simulink model "nav_flocking33"  (R2022b)
settings: Solver=FixedStepAuto  StartTime=0.0  StopTime=10.0  FixedStep=0.01  RelTol=1e-3
values from neighbouring files (symbols this model uses):
  a = 1    [main_flock3.m]    (also in main_flock4.m; params_flocking_ros.m)
  aR = diag([ar; ap; ay])    [main_flock3.m]    (also in main_flock4.m; main_sliding.m)
  Att1 = [2 -2 -15]    [main_flock3.m]    (also in main_flock4.m)
  Att2 = [2 -2 -15]    [main_flock3.m]    (also in main_flock4.m)
  Att3 = [2 -2 -15]    [main_flock3.m]    (also in main_flock4.m)
  b = 1    [main_flock3.m]    (also in main_flock4.m; params_flocking_ros.m)
  c = 1    [main_flock3.m]    (also in main_flock4.m; params_flocking_ros.m)
  c_gammap = 1.2    [main_flock3.m]    (also in main_flock4.m)
  c_gammav = 3.5    [main_flock3.m]    (also in main_flock4.m)
  d = 0.6    [main_flock3.m]    (also in main_flock4.m; params_flocking_ros.m)
  d_prime = 1    [main_flock3.m]    (also in main_flock4.m; params_flocking_ros.m)
  epsilon = 0.1    [main_flock3.m]    (also in main_flock4.m; params_flocking_ros.m)
  h = 0.2    [main_flock3.m]    (also in main_flock4.m; params_flocking_ros.m)
  K1 = diag([k111; k122; k133])    [main_flock3.m]    (also in main_flock4.m; main_sliding.m)
  K2 = diag([k211; k222; k233])    [main_flock3.m]    (also in main_flock4.m; main_sliding.m)
  Ki = diag([Ki1; Ki2; Ki3])    [main_flock3.m]    (also in main_flock4.m; main_sliding.m)
  lam = diag([lam1; lam2; lam3])    [main_flock3.m]    (also in main_flock4.m; main_sliding.m)
  R = 0.15    [main_flock3.m]    (also in main_flock4.m; params_flocking_ros.m)
  vxobs = 0    [main_flock3.m]    (also in main_flock4.m)
  vyobs = 0    [main_flock3.m]    (also in main_flock4.m)
  vzobs = 0    [main_flock3.m]    (also in main_flock4.m)
  X0_1 = [P01 dP01 om01]    [main_flock3.m]    (also in main_flock4.m; main_sliding.m = [P0 dP0 om0])
  X0_2 = [P02 dP02 om02]    [main_flock3.m]    (also in main_flock4.m)
  X0_3 = [P03 dP03 om03]    [main_flock3.m]    (also in main_flock4.m)
  xmax = 2    [main_flock3.m]    (also in main_flock4.m)
  xmin = -2    [main_flock3.m]    (also in main_flock4.m)
  xobs = 0.75    [main_flock3.m]    (also in main_flock4.m)
  yobs = -0.25    [main_flock3.m]    (also in main_flock4.m)
  zobs = 1.7    [main_flock3.m]    (also in main_flock4.m)
undefined symbols (not defined in the file or in its folder): A_Euler
libraries: aerosimlib x3
(part 1 of 2)
settings Model: Creator=root  LastModifiedBy=jonatan_alvarez
settings SolverCC: AlgebraicLoopSolver=TrustRegion
settings DataIOCC: ReturnWorkspaceOutputs=off
settings DebuggingCC: UnconnectedInputMsg=warning  UnconnectedOutputMsg=warning  UnconnectedLineMsg=warning  SFMachineParentedDataDiag=warning  UnderSpecifiedDimensionMsg=warning  ArithmeticOperatorsInVariantConditions=warning
settings ModelReferenceCC: EnableRefExpFcnMdlSchedulingChecks=on
settings SFSimCC: CustomCodeUndefinedFunction=UseInterfaceOnly

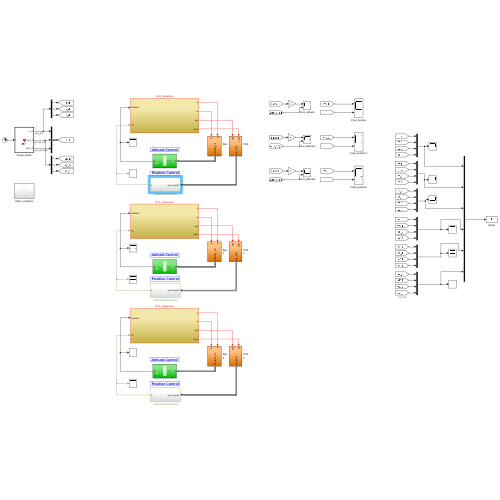
[thumbnail: Simulink's stored preview of the top-level diagram]
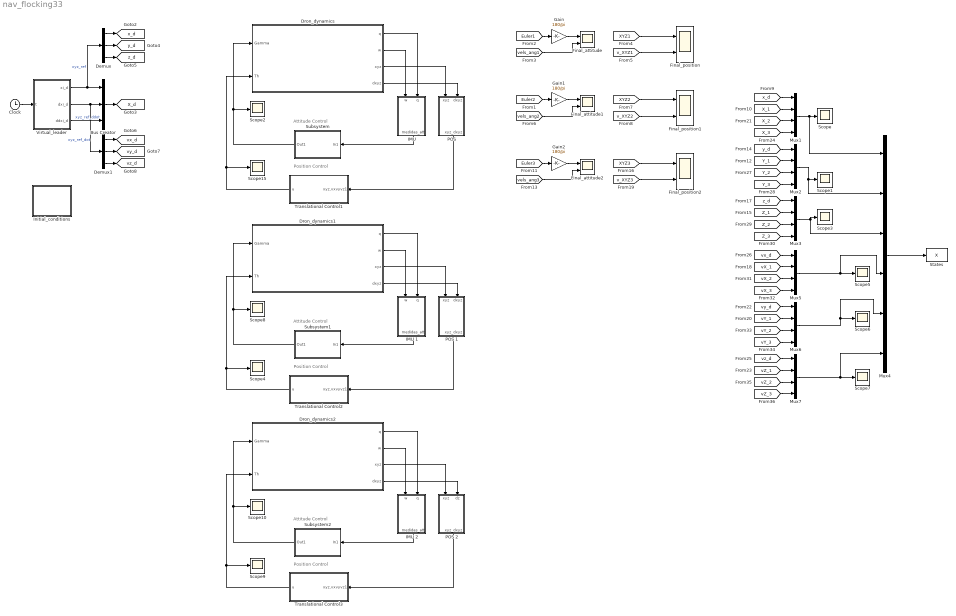
== system nav_flocking33 ==
  note: Position Control
  note: Attitude Control
  note: Position Control
  note: Attitude Control
  note: Position Control
  note: Attitude Control
  Bus Creator : BusCreator  Inputs=3
  Clock : Clock
  Demux : Demux  Outputs=3
  Demux1 : Demux  Outputs=3
  Dron_dynamics : Subsystem
  Dron_dynamics1 : Subsystem
  Dron_dynamics2 : Subsystem
  Final_attitude : Scope  NumInputPorts=2
  Final_attitude1 : Scope  NumInputPorts=2
  Final_attitude2 : Scope  NumInputPorts=2
  Final_position : Scope  NumInputPorts=2
  Final_position1 : Scope  NumInputPorts=2
  Final_position2 : Scope  NumInputPorts=2
  Gain : Gain  Gain=180/pi
  Gain1 : Gain  Gain=180/pi
  Gain2 : Gain  Gain=180/pi
  "IMU " : Subsystem
  IMU 1 : Subsystem
  IMU 2 : Subsystem
  Initial_conditions : Subsystem
  Mux{1..3,5..7} (6 alike) : Mux
  Mux4 : Mux  Inputs=6
  "POS " : Subsystem
  POS 1 : Subsystem
  POS 2 : Subsystem
  Scope{,1..10,15} (12 alike) : Scope
  States : ToWorkspace  VariableName=X  SampleTime=-1
  Subsystem : Subsystem
  Subsystem1 : Subsystem
  Subsystem2 : Subsystem
  Translational Control1 : Subsystem
  Translational Control2 : Subsystem
  Translational Control3 : Subsystem
  Virtual_leader : MATLAB Function  TreatAsAtomicUnit=on
  tag scope: X_d=global, vx_d=global, vy_d=global, vz_d=global, x_d=global, y_d=global, z_d=global
  wires:
  [vels_ang1] -> Final_attitude/2
  [v_XYZ1] -> Final_position/2
  Gain/1 -> Final_attitude/1
  [XYZ1] -> Final_position/1
  [Euler1] -> Gain/1
  Dron_dynamics/2(w) -> "IMU "/1(w)
  Dron_dynamics/4(dxyz) -> "POS "/2(dxyz)
  Bus Creator/1 -> [X_d]
  Virtual_leader/3(ddxi_d) -> Bus Creator/3  "xyz_ref_ddot"
  Dron_dynamics/1(q) -> "IMU "/2(q)
  Subsystem/1(Out1) -> Scope2/1, Dron_dynamics/1(Gamma)
  Dron_dynamics/3(xyz) -> "POS "/1(xyz)
  "POS "/1(xyz_dxyz) -> Translational Control1/1(xyz,vxvyvz1)
  Translational Control1/1(u) -> Scope15/1, Dron_dynamics/2(Th)
  "IMU "/1(medidas_att) -> Subsystem/1(In1)
  Virtual_leader/1(xi_d) -> Demux/1, Bus Creator/1  "xyz_ref"
  Demux/1 -> [x_d]
  Demux/2 -> [y_d]
  Demux/3 -> [z_d]
  [x_d] -> Mux1/1
  [X_1] -> Mux1/2
  Mux2/1 -> Mux4/2, Scope1/1
  [Y_1] -> Mux2/2
  [y_d] -> Mux2/1
  [z_d] -> Mux3/1
  [Z_1] -> Mux3/2
  Mux3/1 -> Scope3/1, Mux4/3
  Mux4/1 -> States/1
  Mux1/1 -> Mux4/1, Scope/1
  Demux1/3 -> [vz_d]
  Demux1/2 -> [vy_d]
  Demux1/1 -> [vx_d]
  Virtual_leader/2(dxi_d) -> Demux1/1, Bus Creator/2  "xyz_ref_dot"
  [vZ_1] -> Mux7/2
  [vz_d] -> Mux7/1
  [vy_d] -> Mux6/1
  [vY_1] -> Mux6/2
  [vX_1] -> Mux5/2
  [vx_d] -> Mux5/1
  Mux5/1 -> Scope5/1, Mux4/4
  Mux6/1 -> Scope6/1, Mux4/5
  Mux7/1 -> Mux4/6, Scope7/1
  Clock/1 -> Virtual_leader/1(t)
  Dron_dynamics1/2(w) -> IMU 1/1(w)
  Dron_dynamics1/4(dxyz) -> POS 1/2(dxyz)
  Dron_dynamics1/3(xyz) -> POS 1/1(xyz)
  POS 1/1(xyz_dxyz) -> Translational Control2/1(xyz,vxvyvz1)
  Dron_dynamics1/1(q) -> IMU 1/2(q)
  Translational Control2/1(u) -> Scope4/1, Dron_dynamics1/2(Th)
  IMU 1/1(medidas_att) -> Subsystem1/1(In1)
  Subsystem1/1(Out1) -> Scope8/1, Dron_dynamics1/1(Gamma)
  Dron_dynamics2/2(w) -> IMU 2/1(w)
  Dron_dynamics2/4(dxyz) -> POS 2/2(dz)
  Dron_dynamics2/3(xyz) -> POS 2/1(xyz)
  POS 2/1(xyz_dxyz) -> Translational Control3/1(xyz,vxvyvz1)
  Dron_dynamics2/1(q) -> IMU 2/2(q)
  Translational Control3/1(u) -> Scope9/1, Dron_dynamics2/2(Th)
  IMU 2/1(medidas_att) -> Subsystem2/1(In1)
  Subsystem2/1(Out1) -> Scope10/1, Dron_dynamics2/1(Gamma)
  [v_XYZ2] -> Final_position1/2
  [Euler2] -> Gain1/1
  Gain1/1 -> Final_attitude1/1
  [XYZ2] -> Final_position1/1
  [vels_ang2] -> Final_attitude1/2
  [v_XYZ3] -> Final_position2/2
  [Euler3] -> Gain2/1
  Gain2/1 -> Final_attitude2/1
  [XYZ3] -> Final_position2/1
  [vels_ang3] -> Final_attitude2/2
  [X_2] -> Mux1/3
  [X_3] -> Mux1/4
  [Y_2] -> Mux2/3
  [Y_3] -> Mux2/4
  [Z_2] -> Mux3/3
  [Z_3] -> Mux3/4
  [vX_2] -> Mux5/3
  [vX_3] -> Mux5/4
  [vY_2] -> Mux6/3
  [vY_3] -> Mux6/4
  [vZ_2] -> Mux7/3
  [vZ_3] -> Mux7/4

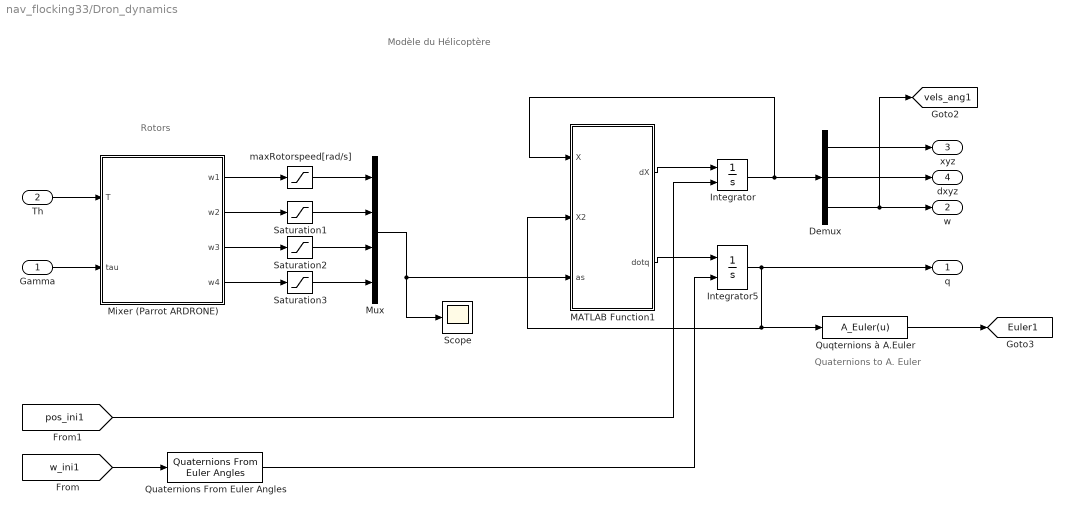
== system nav_flocking33/Dron_dynamics ==
  note: Modèle du Hélicoptère
  note: Rotors
  note: Quaternions to A. Euler
  Gamma : Inport
  Th : Inport  Port=2
  Demux : Demux  Outputs=3
  Integrator : Integrator  InitialConditionSource=external
  Integrator5 : Integrator  InitialConditionSource=external  InitialCondition=[1 0 0 0]
  MATLAB Function1 : MATLAB Function  TreatAsAtomicUnit=on
  Mixer (Parrot ARDRONE) : MATLAB Function  TreatAsAtomicUnit=on
  Mux : Mux
  Quaternions From Euler Angles : aerosimlib/Transformations/Quaternions From Euler Angles
  Quqternions à A.Euler : MATLABFcn  MATLABFcn=A_Euler(u)  OutputDimensions=3
  Saturation1 : Saturate  UpperLimit=1100  LowerLimit=5
  Saturation2 : Saturate  UpperLimit=1100  LowerLimit=5
  Saturation3 : Saturate  UpperLimit=1100  LowerLimit=5
  Scope : Scope
  maxRotorspeed[rad/s] : Saturate  UpperLimit=1100  LowerLimit=5
  q : Outport  VectorParamsAs1DForOutWhenUnconnected=off
  w : Outport  Port=2  VectorParamsAs1DForOutWhenUnconnected=off
  xyz : Outport  Port=3  VectorParamsAs1DForOutWhenUnconnected=off
  dxyz : Outport  Port=4  VectorParamsAs1DForOutWhenUnconnected=off
  tag scope: Euler1=global, vels_ang1=global
  wires:
  [w_ini1] -> Quaternions From Euler Angles/1
  Quqternions à A.Euler/1 -> [Euler1]
  Mixer (Parrot ARDRONE)/4(w4) -> Saturation3/1
  Saturation1/1 -> Mux/2
  Mixer (Parrot ARDRONE)/2(w2) -> Saturation1/1
  Mixer (Parrot ARDRONE)/1(w1) -> maxRotorspeed[rad/s]/1
  maxRotorspeed[rad/s]/1 -> Mux/1
  Saturation3/1 -> Mux/4
  Saturation2/1 -> Mux/3
  Mixer (Parrot ARDRONE)/3(w3) -> Saturation2/1
  Mux/1 -> Scope/1, MATLAB Function1/3(as)
  Integrator5/1 -> MATLAB Function1/2(X2), Quqternions à A.Euler/1, q/1
  MATLAB Function1/1(dX) -> Integrator/1
  MATLAB Function1/2(dotq) -> Integrator5/1
  Quaternions From Euler Angles/1 -> Integrator5/2
  Integrator/1 -> Demux/1, MATLAB Function1/1(X)
  Gamma/1 -> Mixer (Parrot ARDRONE)/2(tau)
  [pos_ini1] -> Integrator/2
  Demux/3 -> [vels_ang1], w/1
  Demux/1 -> xyz/1
  Demux/2 -> dxyz/1
  Th/1 -> Mixer (Parrot ARDRONE)/1(T)

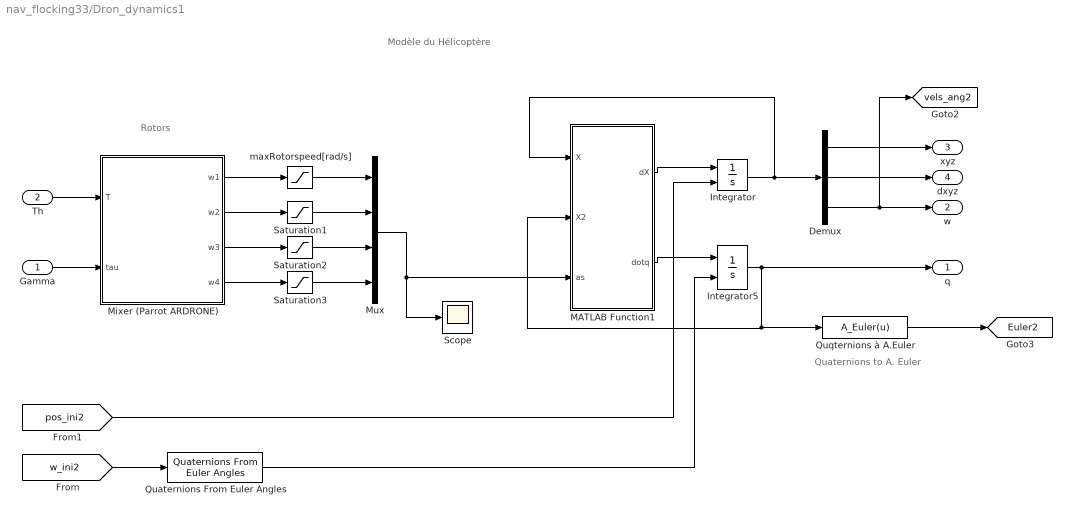
== system nav_flocking33/Dron_dynamics1 ==
  note: Modèle du Hélicoptère
  note: Rotors
  note: Quaternions to A. Euler
  Gamma : Inport
  Th : Inport  Port=2
  Demux : Demux  Outputs=3
  Integrator : Integrator  InitialConditionSource=external
  Integrator5 : Integrator  InitialConditionSource=external  InitialCondition=[1 0 0 0]
  MATLAB Function1 : MATLAB Function  TreatAsAtomicUnit=on
  Mixer (Parrot ARDRONE) : MATLAB Function  TreatAsAtomicUnit=on
  Mux : Mux
  Quaternions From Euler Angles : aerosimlib/Transformations/Quaternions From Euler Angles
  Quqternions à A.Euler : MATLABFcn  MATLABFcn=A_Euler(u)  OutputDimensions=3
  Saturation1 : Saturate  UpperLimit=1100  LowerLimit=5
  Saturation2 : Saturate  UpperLimit=1100  LowerLimit=5
  Saturation3 : Saturate  UpperLimit=1100  LowerLimit=5
  Scope : Scope
  maxRotorspeed[rad/s] : Saturate  UpperLimit=1100  LowerLimit=5
  q : Outport  VectorParamsAs1DForOutWhenUnconnected=off
  w : Outport  Port=2  VectorParamsAs1DForOutWhenUnconnected=off
  xyz : Outport  Port=3  VectorParamsAs1DForOutWhenUnconnected=off
  dxyz : Outport  Port=4  VectorParamsAs1DForOutWhenUnconnected=off
  tag scope: Euler2=global, vels_ang2=global
  wires:
  [w_ini2] -> Quaternions From Euler Angles/1
  Quqternions à A.Euler/1 -> [Euler2]
  Mixer (Parrot ARDRONE)/4(w4) -> Saturation3/1
  Saturation1/1 -> Mux/2
  Mixer (Parrot ARDRONE)/2(w2) -> Saturation1/1
  Mixer (Parrot ARDRONE)/1(w1) -> maxRotorspeed[rad/s]/1
  maxRotorspeed[rad/s]/1 -> Mux/1
  Saturation3/1 -> Mux/4
  Saturation2/1 -> Mux/3
  Mixer (Parrot ARDRONE)/3(w3) -> Saturation2/1
  Mux/1 -> Scope/1, MATLAB Function1/3(as)
  Integrator5/1 -> MATLAB Function1/2(X2), Quqternions à A.Euler/1, q/1
  MATLAB Function1/1(dX) -> Integrator/1
  MATLAB Function1/2(dotq) -> Integrator5/1
  Quaternions From Euler Angles/1 -> Integrator5/2
  Integrator/1 -> Demux/1, MATLAB Function1/1(X)
  Gamma/1 -> Mixer (Parrot ARDRONE)/2(tau)
  [pos_ini2] -> Integrator/2
  Demux/3 -> [vels_ang2], w/1
  Demux/1 -> xyz/1
  Demux/2 -> dxyz/1
  Th/1 -> Mixer (Parrot ARDRONE)/1(T)

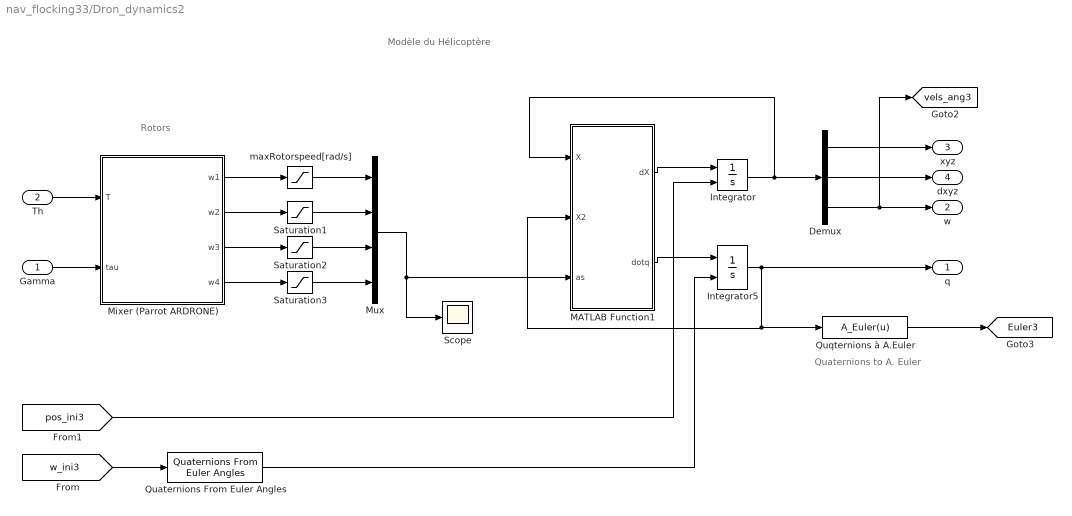
== system nav_flocking33/Dron_dynamics2 ==
  note: Modèle du Hélicoptère
  note: Rotors
  note: Quaternions to A. Euler
  Gamma : Inport
  Th : Inport  Port=2
  Demux : Demux  Outputs=3
  Integrator : Integrator  InitialConditionSource=external
  Integrator5 : Integrator  InitialConditionSource=external  InitialCondition=[1 0 0 0]
  MATLAB Function1 : MATLAB Function  TreatAsAtomicUnit=on
  Mixer (Parrot ARDRONE) : MATLAB Function  TreatAsAtomicUnit=on
  Mux : Mux
  Quaternions From Euler Angles : aerosimlib/Transformations/Quaternions From Euler Angles
  Quqternions à A.Euler : MATLABFcn  MATLABFcn=A_Euler(u)  OutputDimensions=3
  Saturation1 : Saturate  UpperLimit=1100  LowerLimit=5
  Saturation2 : Saturate  UpperLimit=1100  LowerLimit=5
  Saturation3 : Saturate  UpperLimit=1100  LowerLimit=5
  Scope : Scope
  maxRotorspeed[rad/s] : Saturate  UpperLimit=1100  LowerLimit=5
  q : Outport  VectorParamsAs1DForOutWhenUnconnected=off
  w : Outport  Port=2  VectorParamsAs1DForOutWhenUnconnected=off
  xyz : Outport  Port=3  VectorParamsAs1DForOutWhenUnconnected=off
  dxyz : Outport  Port=4  VectorParamsAs1DForOutWhenUnconnected=off
  tag scope: Euler3=global, vels_ang3=global
  wires:
  [w_ini3] -> Quaternions From Euler Angles/1
  Quqternions à A.Euler/1 -> [Euler3]
  Mixer (Parrot ARDRONE)/4(w4) -> Saturation3/1
  Saturation1/1 -> Mux/2
  Mixer (Parrot ARDRONE)/2(w2) -> Saturation1/1
  Mixer (Parrot ARDRONE)/1(w1) -> maxRotorspeed[rad/s]/1
  maxRotorspeed[rad/s]/1 -> Mux/1
  Saturation3/1 -> Mux/4
  Saturation2/1 -> Mux/3
  Mixer (Parrot ARDRONE)/3(w3) -> Saturation2/1
  Mux/1 -> Scope/1, MATLAB Function1/3(as)
  Integrator5/1 -> MATLAB Function1/2(X2), Quqternions à A.Euler/1, q/1
  MATLAB Function1/1(dX) -> Integrator/1
  MATLAB Function1/2(dotq) -> Integrator5/1
  Quaternions From Euler Angles/1 -> Integrator5/2
  Integrator/1 -> Demux/1, MATLAB Function1/1(X)
  Gamma/1 -> Mixer (Parrot ARDRONE)/2(tau)
  [pos_ini3] -> Integrator/2
  Demux/3 -> [vels_ang3], w/1
  Demux/1 -> xyz/1
  Demux/2 -> dxyz/1
  Th/1 -> Mixer (Parrot ARDRONE)/1(T)

== system nav_flocking33/IMU  ==
  w : Inport
  q : Inport  Port=2
  Bus Creator : BusCreator  Inputs=4
  Display : Display
  Integrator : Integrator
  Scope : Scope
  q_e : Subsystem
  medidas_att : Outport  VectorParamsAs1DForOutWhenUnconnected=off
  wires:
  [q_d1] -> q_e/1(q1)
  q/1 -> Bus Creator/1, q_e/2(Q2)
  w/1 -> Bus Creator/3
  Integrator/1 -> Display/1, Bus Creator/4
  Bus Creator/1 -> medidas_att/1
  q_e/1(qxQ) -> Integrator/1, Scope/1, Bus Creator/2

== system nav_flocking33/IMU 1 ==
  w : Inport
  q : Inport  Port=2
  Bus Creator : BusCreator  Inputs=4
  Display : Display
  Integrator : Integrator
  Scope : Scope
  q_e : Subsystem
  medidas_att : Outport  VectorParamsAs1DForOutWhenUnconnected=off
  wires:
  [q_d2] -> q_e/1(q1)
  q/1 -> Bus Creator/1, q_e/2(Q2)
  w/1 -> Bus Creator/3
  Integrator/1 -> Display/1, Bus Creator/4
  Bus Creator/1 -> medidas_att/1
  q_e/1(qxQ) -> Integrator/1, Scope/1, Bus Creator/2

== system nav_flocking33/IMU 2 ==
  w : Inport
  q : Inport  Port=2
  Bus Creator : BusCreator  Inputs=4
  Display : Display
  Integrator : Integrator
  Scope : Scope
  q_e : Subsystem
  medidas_att : Outport  VectorParamsAs1DForOutWhenUnconnected=off
  wires:
  [q_d3] -> q_e/1(q1)
  q/1 -> Bus Creator/1, q_e/2(Q2)
  w/1 -> Bus Creator/3
  Integrator/1 -> Display/1, Bus Creator/4
  Bus Creator/1 -> medidas_att/1
  q_e/1(qxQ) -> Integrator/1, Scope/1, Bus Creator/2

== system nav_flocking33/Initial_conditions ==
  "phi, theta,psi Condition Initiale" : Constant  Value=[Att1]*pi/180
  "phi, theta,psi Condition Initiale1" : Constant  Value=X0_1
  "phi, theta,psi Condition Initiale2" : Constant  Value=[Att2]*pi/180
  "phi, theta,psi Condition Initiale3" : Constant  Value=X0_2
  "phi, theta,psi Condition Initiale4" : Constant  Value=[Att3]*pi/180
  "phi, theta,psi Condition Initiale5" : Constant  Value=X0_3
  tag scope: pos_ini1=global, pos_ini2=global, pos_ini3=global, w_ini1=global, w_ini2=global, w_ini3=global
  wires:
  "phi, theta,psi Condition Initiale1"/1 -> [pos_ini1]
  "phi, theta,psi Condition Initiale"/1 -> [w_ini1]
  "phi, theta,psi Condition Initiale2"/1 -> [w_ini2]
  "phi, theta,psi Condition Initiale3"/1 -> [pos_ini2]
  "phi, theta,psi Condition Initiale4"/1 -> [w_ini3]
  "phi, theta,psi Condition Initiale5"/1 -> [pos_ini3]

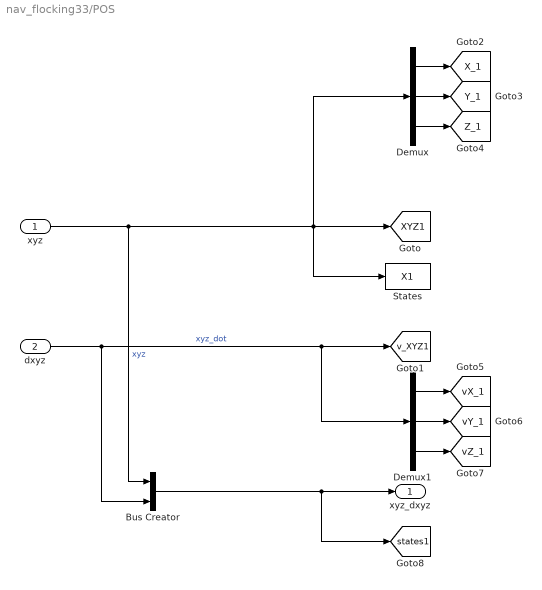
== system nav_flocking33/POS  ==
  xyz : Inport
  dxyz : Inport  Port=2
  Bus Creator : BusCreator  Inputs=2
  Demux : Demux  Outputs=3
  Demux1 : Demux  Outputs=3
  States : ToWorkspace  VariableName=X1  SampleTime=-1
  xyz_dxyz : Outport  VectorParamsAs1DForOutWhenUnconnected=off
  tag scope: XYZ1=global, X_1=global, Y_1=global, Z_1=global, states1=global, vX_1=global, vY_1=global, vZ_1=global, v_XYZ1=global
  wires:
  xyz/1 -> Bus Creator/1, States/1, Demux/1, [XYZ1]  "xyz"
  dxyz/1 -> Bus Creator/2, Demux1/1, [v_XYZ1]  "xyz_dot"
  Demux/1 -> [X_1]
  Demux/2 -> [Y_1]
  Demux/3 -> [Z_1]
  Demux1/3 -> [vZ_1]
  Demux1/2 -> [vY_1]
  Demux1/1 -> [vX_1]
  Bus Creator/1 -> [states1], xyz_dxyz/1

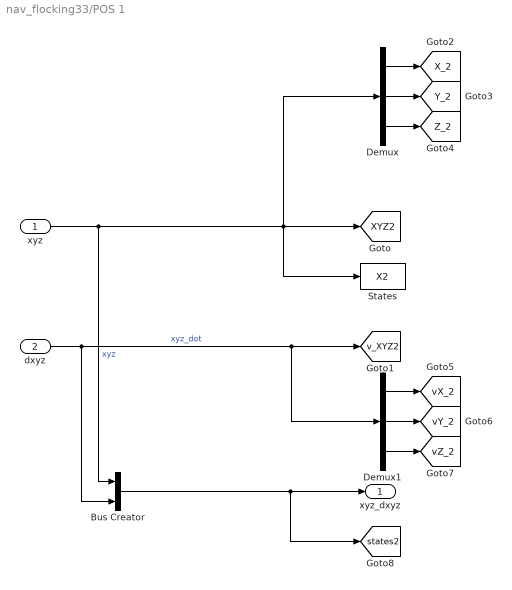
== system nav_flocking33/POS 1 ==
  xyz : Inport
  dxyz : Inport  Port=2
  Bus Creator : BusCreator  Inputs=2
  Demux : Demux  Outputs=3
  Demux1 : Demux  Outputs=3
  States : ToWorkspace  VariableName=X2  SampleTime=-1
  xyz_dxyz : Outport  VectorParamsAs1DForOutWhenUnconnected=off
  tag scope: XYZ2=global, X_2=global, Y_2=global, Z_2=global, states2=global, vX_2=global, vY_2=global, vZ_2=global, v_XYZ2=global
  wires:
  xyz/1 -> Bus Creator/1, States/1, Demux/1, [XYZ2]  "xyz"
  dxyz/1 -> Bus Creator/2, Demux1/1, [v_XYZ2]  "xyz_dot"
  Demux/1 -> [X_2]
  Demux/2 -> [Y_2]
  Demux/3 -> [Z_2]
  Bus Creator/1 -> [states2], xyz_dxyz/1
  Demux1/3 -> [vZ_2]
  Demux1/2 -> [vY_2]
  Demux1/1 -> [vX_2]

== system nav_flocking33/POS 2 ==
  xyz : Inport
  dz : Inport  Port=2
  Bus Creator : BusCreator  Inputs=2
  Demux : Demux  Outputs=3
  Demux1 : Demux  Outputs=3
  States : ToWorkspace  VariableName=X3  SampleTime=-1
  xyz_dxyz : Outport  VectorParamsAs1DForOutWhenUnconnected=off
  tag scope: XYZ3=global, X_3=global, Y_3=global, Z_3=global, states3=global, vX_3=global, vY_3=global, vZ_3=global, v_XYZ3=global
  wires:
  xyz/1 -> Bus Creator/1, States/1, Demux/1, [XYZ3]  "xyz"
  dz/1 -> Bus Creator/2, Demux1/1, [v_XYZ3]  "xyz_dot"
  Demux/1 -> [X_3]
  Demux/2 -> [Y_3]
  Demux/3 -> [Z_3]
  Bus Creator/1 -> [states3], xyz_dxyz/1
  Demux1/3 -> [vZ_3]
  Demux1/2 -> [vY_3]
  Demux1/1 -> [vX_3]

== system nav_flocking33/Subsystem ==
  In1 : Inport
  Scope : Scope
  Sliding mode (quaternions) : MATLAB Function  Description=Integral quaternion Sliding mode control  TreatAsAtomicUnit=on
  Out1 : Outport  VectorParamsAs1DForOutWhenUnconnected=off
  wires:
  In1/1 -> Sliding mode (quaternions)/1(qwe)
  Sliding mode (quaternions)/1(Gamma) -> Out1/1
  Sliding mode (quaternions)/2(s) -> Scope/1

== system nav_flocking33/Subsystem1 ==
  In1 : Inport
  Scope : Scope
  Sliding mode (quaternions) : MATLAB Function  Description=Integral quaternion Sliding mode control  TreatAsAtomicUnit=on
  Out1 : Outport  VectorParamsAs1DForOutWhenUnconnected=off
  wires:
  In1/1 -> Sliding mode (quaternions)/1(qwe)
  Sliding mode (quaternions)/1(Gamma) -> Out1/1
  Sliding mode (quaternions)/2(s) -> Scope/1

== system nav_flocking33/Subsystem2 ==
  In1 : Inport
  Scope : Scope
  Sliding mode (quaternions) : MATLAB Function  Description=Integral quaternion Sliding mode control  TreatAsAtomicUnit=on
  Out1 : Outport  VectorParamsAs1DForOutWhenUnconnected=off
  wires:
  In1/1 -> Sliding mode (quaternions)/1(qwe)
  Sliding mode (quaternions)/1(Gamma) -> Out1/1
  Sliding mode (quaternions)/2(s) -> Scope/1

== system nav_flocking33/Translational Control1 ==
  xyz,vxvyvz1 : Inport
  Flocking1 : Subsystem
  Scope2 : Scope
  Scope3 : Scope
  to_desired_angles : MATLAB Function  TreatAsAtomicUnit=on
  u : Outport  VectorParamsAs1DForOutWhenUnconnected=off
  tag scope: q_d1=global, u_1=global
  wires:
  to_desired_angles/2(Uz) -> u/1
  to_desired_angles/1(cq_d) -> Scope2/1, [q_d1]
  [X_d] -> Flocking1/1(ref)
  xyz,vxvyvz1/1 -> Flocking1/2(state)
  Flocking1/1(U_i) -> [u_1], Scope3/1, to_desired_angles/1(Gamma)
  [states2] -> Flocking1/3(statej)
  [states3] -> Flocking1/4(statek)

== system nav_flocking33/Translational Control2 ==
  xyz,vxvyvz1 : Inport
  Flocking1 : Subsystem
  Scope2 : Scope
  Scope3 : Scope
  to_desired_angles : MATLAB Function  TreatAsAtomicUnit=on
  u : Outport  VectorParamsAs1DForOutWhenUnconnected=off
  tag scope: q_d2=global, u_2=global
  wires:
  to_desired_angles/2(Uz) -> u/1
  to_desired_angles/1(cq_d) -> Scope2/1, [q_d2]
  [X_d] -> Flocking1/1(ref)
  xyz,vxvyvz1/1 -> Flocking1/2(state)
  Flocking1/1(U_i) -> [u_2], Scope3/1, to_desired_angles/1(Gamma)
  [states1] -> Flocking1/3(statej)
  [states3] -> Flocking1/4(statek)

== system nav_flocking33/Translational Control3 ==
  xyz,vxvyvz1 : Inport
  Flocking1 : Subsystem
  Scope2 : Scope
  Scope3 : Scope
  to_desired_angles : MATLAB Function  TreatAsAtomicUnit=on
  u : Outport  VectorParamsAs1DForOutWhenUnconnected=off
  tag scope: q_d3=global, u_3=global
  wires:
  to_desired_angles/2(Uz) -> u/1
  to_desired_angles/1(cq_d) -> Scope2/1, [q_d3]
  [X_d] -> Flocking1/1(ref)
  xyz,vxvyvz1/1 -> Flocking1/2(state)
  Flocking1/1(U_i) -> [u_3], Scope3/1, to_desired_angles/1(Gamma)
  [states1] -> Flocking1/3(statej)
  [states2] -> Flocking1/4(statek)

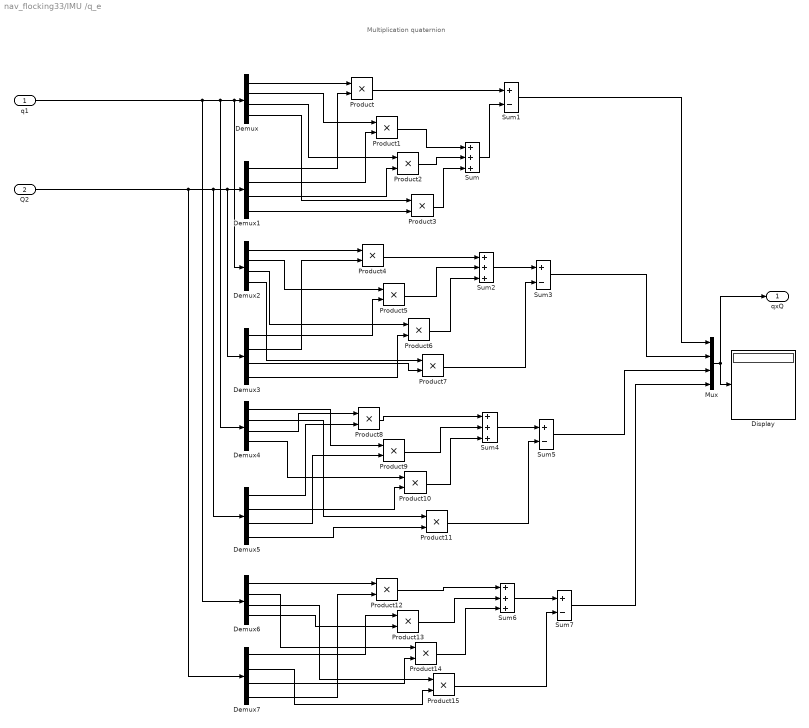
== system nav_flocking33/IMU /q_e ==
  note: Multiplication quaternion
  q1 : Inport
  Q2 : Inport  Port=2
  Demux{,1..7} (8 alike) : Demux
  Display : Display
  Mux : Mux
  Product{,1..15} (16 alike) : Product  RndMeth=Zero
  Sum{,2,4,6} (4 alike) : Sum  Inputs=+++
  Sum{1,3,5,7} (4 alike) : Sum  Inputs=+-
  qxQ : Outport  VectorParamsAs1DForOutWhenUnconnected=off
  wires:
  q1/1 -> Demux/1, Demux2/1, Demux4/1, Demux6/1
  Q2/1 -> Demux1/1, Demux3/1, Demux5/1, Demux7/1
  Demux/1 -> Product/1
  Demux1/1 -> Product/2
  Demux/2 -> Product1/1
  Demux1/2 -> Product1/2
  Demux/3 -> Product2/1
  Demux1/3 -> Product2/2
  Demux/4 -> Product3/1
  Demux1/4 -> Product3/2
  Product1/1 -> Sum/1
  Product2/1 -> Sum/2
  Product3/1 -> Sum/3
  Sum/1 -> Sum1/2
  Product/1 -> Sum1/1
  Demux2/1 -> Product4/1
  Demux3/2 -> Product4/2
  Demux2/2 -> Product5/1
  Demux3/1 -> Product5/2
  Demux2/3 -> Product6/1
  Demux3/4 -> Product6/2
  Demux2/4 -> Product7/1
  Demux3/3 -> Product7/2
  Product4/1 -> Sum2/1
  Product5/1 -> Sum2/2
  Product6/1 -> Sum2/3
  Sum2/1 -> Sum3/1
  Product7/1 -> Sum3/2
  Demux4/3 -> Product8/1
  Demux5/1 -> Product8/2
  Demux4/1 -> Product9/1
  Demux5/3 -> Product9/2
  Demux4/4 -> Product10/1
  Demux5/2 -> Product10/2
  Demux5/4 -> Product11/2
  Demux4/2 -> Product11/1
  Sum4/1 -> Sum5/1
  Product11/1 -> Sum5/2
  Product8/1 -> Sum4/1
  Product9/1 -> Sum4/2
  Product10/1 -> Sum4/3
  Demux6/1 -> Product12/1
  Demux7/1 -> Product13/1
  Demux6/2 -> Product14/1
  Demux7/4 -> Product12/2
  Demux6/4 -> Product13/2
  Demux7/3 -> Product14/2
  Demux6/3 -> Product15/1
  Demux7/2 -> Product15/2
  Sum6/1 -> Sum7/1
  Product15/1 -> Sum7/2
  Product12/1 -> Sum6/1
  Product13/1 -> Sum6/2
  Product14/1 -> Sum6/3
  Sum1/1 -> Mux/1
  Sum3/1 -> Mux/2
  Sum5/1 -> Mux/3
  Sum7/1 -> Mux/4
  Mux/1 -> Display/1, qxQ/1

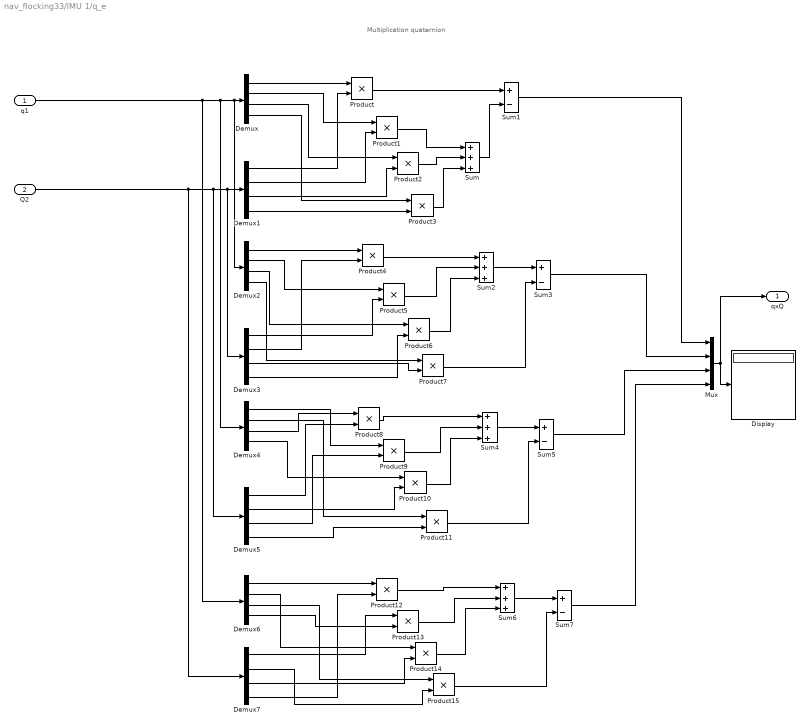
== system nav_flocking33/IMU 1/q_e ==
  note: Multiplication quaternion
  q1 : Inport
  Q2 : Inport  Port=2
  Demux{,1..7} (8 alike) : Demux
  Display : Display
  Mux : Mux
  Product{,1..15} (16 alike) : Product  RndMeth=Zero
  Sum{,2,4,6} (4 alike) : Sum  Inputs=+++
  Sum{1,3,5,7} (4 alike) : Sum  Inputs=+-
  qxQ : Outport  VectorParamsAs1DForOutWhenUnconnected=off
  wires:
  q1/1 -> Demux/1, Demux2/1, Demux4/1, Demux6/1
  Q2/1 -> Demux1/1, Demux3/1, Demux5/1, Demux7/1
  Demux/1 -> Product/1
  Demux1/1 -> Product/2
  Demux/2 -> Product1/1
  Demux1/2 -> Product1/2
  Demux/3 -> Product2/1
  Demux1/3 -> Product2/2
  Demux/4 -> Product3/1
  Demux1/4 -> Product3/2
  Product1/1 -> Sum/1
  Product2/1 -> Sum/2
  Product3/1 -> Sum/3
  Sum/1 -> Sum1/2
  Product/1 -> Sum1/1
  Demux2/1 -> Product4/1
  Demux3/2 -> Product4/2
  Demux2/2 -> Product5/1
  Demux3/1 -> Product5/2
  Demux2/3 -> Product6/1
  Demux3/4 -> Product6/2
  Demux2/4 -> Product7/1
  Demux3/3 -> Product7/2
  Product4/1 -> Sum2/1
  Product5/1 -> Sum2/2
  Product6/1 -> Sum2/3
  Sum2/1 -> Sum3/1
  Product7/1 -> Sum3/2
  Demux4/3 -> Product8/1
  Demux5/1 -> Product8/2
  Demux4/1 -> Product9/1
  Demux5/3 -> Product9/2
  Demux4/4 -> Product10/1
  Demux5/2 -> Product10/2
  Demux5/4 -> Product11/2
  Demux4/2 -> Product11/1
  Sum4/1 -> Sum5/1
  Product11/1 -> Sum5/2
  Product8/1 -> Sum4/1
  Product9/1 -> Sum4/2
  Product10/1 -> Sum4/3
  Demux6/1 -> Product12/1
  Demux7/1 -> Product13/1
  Demux6/2 -> Product14/1
  Demux7/4 -> Product12/2
  Demux6/4 -> Product13/2
  Demux7/3 -> Product14/2
  Demux6/3 -> Product15/1
  Demux7/2 -> Product15/2
  Sum6/1 -> Sum7/1
  Product15/1 -> Sum7/2
  Product12/1 -> Sum6/1
  Product13/1 -> Sum6/2
  Product14/1 -> Sum6/3
  Sum1/1 -> Mux/1
  Sum3/1 -> Mux/2
  Sum5/1 -> Mux/3
  Sum7/1 -> Mux/4
  Mux/1 -> Display/1, qxQ/1

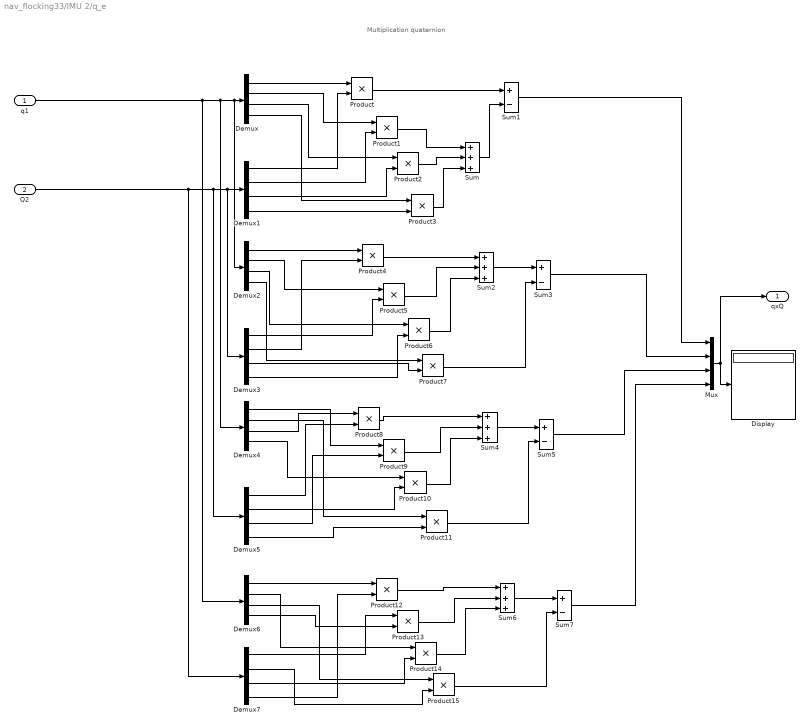
== system nav_flocking33/IMU 2/q_e ==
  note: Multiplication quaternion
  q1 : Inport
  Q2 : Inport  Port=2
  Demux{,1..7} (8 alike) : Demux
  Display : Display
  Mux : Mux
  Product{,1..15} (16 alike) : Product  RndMeth=Zero
  Sum{,2,4,6} (4 alike) : Sum  Inputs=+++
  Sum{1,3,5,7} (4 alike) : Sum  Inputs=+-
  qxQ : Outport  VectorParamsAs1DForOutWhenUnconnected=off
  wires:
  q1/1 -> Demux/1, Demux2/1, Demux4/1, Demux6/1
  Q2/1 -> Demux1/1, Demux3/1, Demux5/1, Demux7/1
  Demux/1 -> Product/1
  Demux1/1 -> Product/2
  Demux/2 -> Product1/1
  Demux1/2 -> Product1/2
  Demux/3 -> Product2/1
  Demux1/3 -> Product2/2
  Demux/4 -> Product3/1
  Demux1/4 -> Product3/2
  Product1/1 -> Sum/1
  Product2/1 -> Sum/2
  Product3/1 -> Sum/3
  Sum/1 -> Sum1/2
  Product/1 -> Sum1/1
  Demux2/1 -> Product4/1
  Demux3/2 -> Product4/2
  Demux2/2 -> Product5/1
  Demux3/1 -> Product5/2
  Demux2/3 -> Product6/1
  Demux3/4 -> Product6/2
  Demux2/4 -> Product7/1
  Demux3/3 -> Product7/2
  Product4/1 -> Sum2/1
  Product5/1 -> Sum2/2
  Product6/1 -> Sum2/3
  Sum2/1 -> Sum3/1
  Product7/1 -> Sum3/2
  Demux4/3 -> Product8/1
  Demux5/1 -> Product8/2
  Demux4/1 -> Product9/1
  Demux5/3 -> Product9/2
  Demux4/4 -> Product10/1
  Demux5/2 -> Product10/2
  Demux5/4 -> Product11/2
  Demux4/2 -> Product11/1
  Sum4/1 -> Sum5/1
  Product11/1 -> Sum5/2
  Product8/1 -> Sum4/1
  Product9/1 -> Sum4/2
  Product10/1 -> Sum4/3
  Demux6/1 -> Product12/1
  Demux7/1 -> Product13/1
  Demux6/2 -> Product14/1
  Demux7/4 -> Product12/2
  Demux6/4 -> Product13/2
  Demux7/3 -> Product14/2
  Demux6/3 -> Product15/1
  Demux7/2 -> Product15/2
  Sum6/1 -> Sum7/1
  Product15/1 -> Sum7/2
  Product12/1 -> Sum6/1
  Product13/1 -> Sum6/2
  Product14/1 -> Sum6/3
  Sum1/1 -> Mux/1
  Sum3/1 -> Mux/2
  Sum5/1 -> Mux/3
  Sum7/1 -> Mux/4
  Mux/1 -> Display/1, qxQ/1

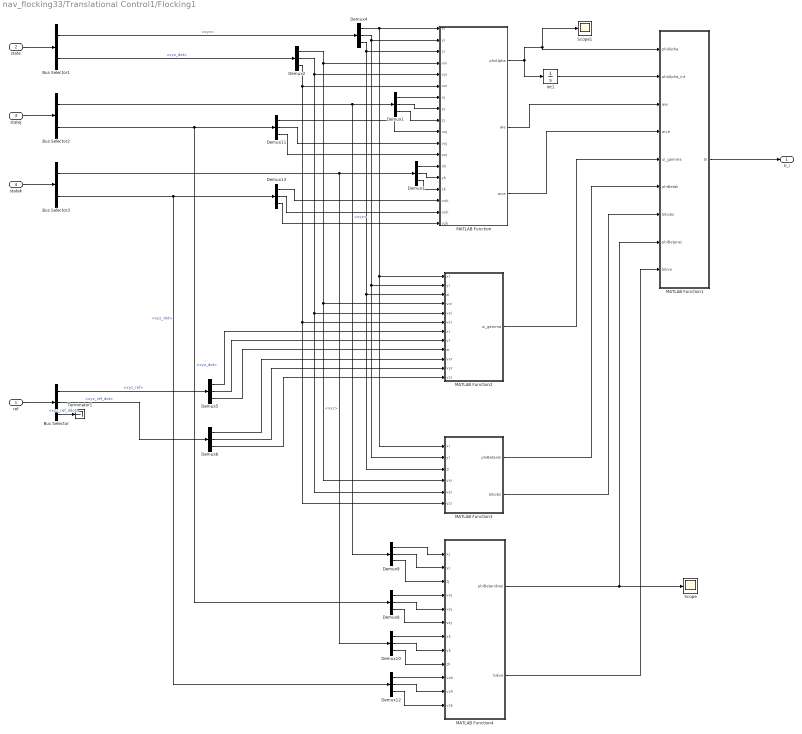
== system nav_flocking33/Translational Control1/Flocking1 ==
  ref : Inport
  state : Inport  Port=2
  statej : Inport  Port=3
  statek : Inport  Port=4
  Bus Selector : BusSelector  OutputSignals=xyz_ref,xyz_ref_dot,xyz_ref_ddot
  Bus Selector1 : BusSelector  OutputSignals=xyz,xyz_dot
  Bus Selector2 : BusSelector  OutputSignals=xyz,xyz_dot
  Bus Selector3 : BusSelector  OutputSignals=xyz,xyz_dot
  Demux{1..6,8..13} (12 alike) : Demux  Outputs=3
  MATLAB Function : MATLAB Function  TreatAsAtomicUnit=on
  MATLAB Function1 : MATLAB Function  TreatAsAtomicUnit=on
  MATLAB Function2 : MATLAB Function  TreatAsAtomicUnit=on
  MATLAB Function3 : MATLAB Function  TreatAsAtomicUnit=on
  MATLAB Function4 : MATLAB Function  TreatAsAtomicUnit=on
  Scope : Scope
  Scope1 : Scope
  Terminator1 : Terminator
  int1 : Integrator
  U_i : Outport  VectorParamsAs1DForOutWhenUnconnected=off
  wires:
  ref/1 -> Bus Selector/1
  state/1 -> Bus Selector1/1
  Bus Selector/2 -> Demux6/1  "<xyz_ref_dot>"
  Bus Selector/1 -> Demux5/1  "<xyz_ref>"
  Bus Selector1/1 -> Demux4/1  "<xyz>"
  Demux6/1 -> MATLAB Function2/10(vxr)
  Demux6/2 -> MATLAB Function2/11(vyr)
  statej/1 -> Bus Selector2/1
  Bus Selector2/1 -> Demux9/1, Demux1/1  "<xyz>"
  Demux4/1 -> MATLAB Function3/1(xi), MATLAB Function2/1(xi), MATLAB Function/1(xi)
  Demux4/2 -> MATLAB Function3/2(yi), MATLAB Function2/2(yi), MATLAB Function/2(yi)
  Demux1/1 -> MATLAB Function/7(xj)
  Demux1/2 -> MATLAB Function/8(yj)
  Bus Selector2/2 -> Demux8/1, Demux11/1  "<xyz_dot>"
  int1/1 -> MATLAB Function1/2(phiAlpha_int)
  MATLAB Function2/1(ui_gamma) -> MATLAB Function1/5(ui_gamma)
  statek/1 -> Bus Selector3/1
  Bus Selector3/2 -> Demux12/1, Demux13/1  "<xyz_dot>"
  Demux3/1 -> MATLAB Function/13(xk)
  Demux3/2 -> MATLAB Function/14(yk)
  Bus Selector3/1 -> Demux10/1, Demux3/1  "<xyz>"
  Demux9/1 -> MATLAB Function4/1(xj)
  Demux9/2 -> MATLAB Function4/2(yj)
  Demux10/1 -> MATLAB Function4/7(xk)
  Demux10/2 -> MATLAB Function4/8(yk)
  MATLAB Function/1(phiAlpha) -> int1/1, Scope1/1, MATLAB Function1/1(phiAlpha)
  Demux5/1 -> MATLAB Function2/7(xr)
  Demux5/2 -> MATLAB Function2/8(yr)
  Bus Selector1/2 -> Demux2/1  "<xyz_dot>"
  Demux4/3 -> MATLAB Function3/3(zi), MATLAB Function2/3(zi), MATLAB Function/3(zi)
  Demux3/3 -> MATLAB Function/15(zk)
  Demux5/3 -> MATLAB Function2/9(zr)
  Demux6/3 -> MATLAB Function2/12(vzr)
  MATLAB Function1/1(Ui) -> U_i/1
  Demux2/1 -> MATLAB Function/4(vxi), MATLAB Function2/4(vxi), MATLAB Function3/4(vxi)
  Demux2/2 -> MATLAB Function/5(vyi), MATLAB Function3/5(vyi), MATLAB Function2/5(vyi)
  Demux2/3 -> MATLAB Function/6(vzi), MATLAB Function3/6(vzi), MATLAB Function2/6(vzi)
  Demux1/3 -> MATLAB Function/9(zj)
  Demux11/1 -> MATLAB Function/10(vxj)
  Demux11/2 -> MATLAB Function/11(vyj)
  Demux11/3 -> MATLAB Function/12(vzj)
  Demux13/1 -> MATLAB Function/16(vxk)
  Demux13/2 -> MATLAB Function/17(vyk)
  Demux13/3 -> MATLAB Function/18(vzk)
  MATLAB Function/3(aive) -> MATLAB Function1/4(aive)
  Demux9/3 -> MATLAB Function4/3(zj)
  Demux10/3 -> MATLAB Function4/9(zk)
  MATLAB Function4/1(phiBetaniknei) -> Scope/1, MATLAB Function1/8(phiBetanei)
  Bus Selector/3 -> Terminator1/1  "<xyz_ref_ddot>"
  Demux8/1 -> MATLAB Function4/4(vxj)
  Demux8/2 -> MATLAB Function4/5(vyj)
  Demux8/3 -> MATLAB Function4/6(vzj)
  Demux12/1 -> MATLAB Function4/10(vxk)
  Demux12/2 -> MATLAB Function4/11(vyk)
  Demux12/3 -> MATLAB Function4/12(vzk)
  MATLAB Function4/2(bikve) -> MATLAB Function1/9(bikve)
  MATLAB Function3/1(phiBetanik) -> MATLAB Function1/6(phiBetak)
  MATLAB Function3/2(bikobs) -> MATLAB Function1/7(bikobs)
  MATLAB Function/2(aie) -> MATLAB Function1/3(aie)

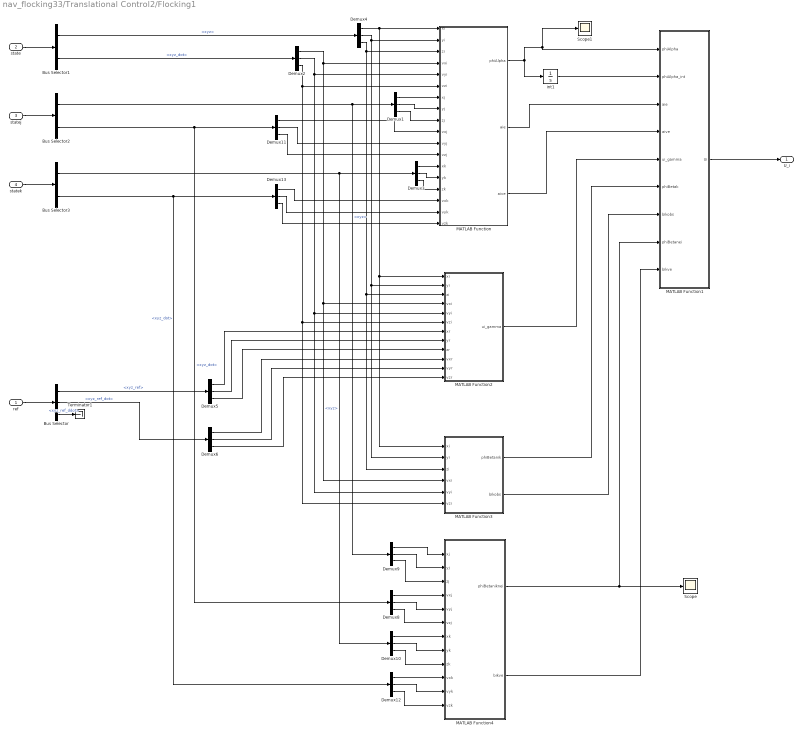
== system nav_flocking33/Translational Control2/Flocking1 ==
  ref : Inport
  state : Inport  Port=2
  statej : Inport  Port=3
  statek : Inport  Port=4
  Bus Selector : BusSelector  OutputSignals=xyz_ref,xyz_ref_dot,xyz_ref_ddot
  Bus Selector1 : BusSelector  OutputSignals=xyz,xyz_dot
  Bus Selector2 : BusSelector  OutputSignals=xyz,xyz_dot
  Bus Selector3 : BusSelector  OutputSignals=xyz,xyz_dot
  Demux{1..6,8..13} (12 alike) : Demux  Outputs=3
  MATLAB Function : MATLAB Function  TreatAsAtomicUnit=on
  MATLAB Function1 : MATLAB Function  TreatAsAtomicUnit=on
  MATLAB Function2 : MATLAB Function  TreatAsAtomicUnit=on
  MATLAB Function3 : MATLAB Function  TreatAsAtomicUnit=on
  MATLAB Function4 : MATLAB Function  TreatAsAtomicUnit=on
  Scope : Scope
  Scope1 : Scope
  Terminator1 : Terminator
  int1 : Integrator
  U_i : Outport  VectorParamsAs1DForOutWhenUnconnected=off
  wires:
  ref/1 -> Bus Selector/1
  state/1 -> Bus Selector1/1
  Bus Selector/2 -> Demux6/1  "<xyz_ref_dot>"
  Bus Selector/1 -> Demux5/1  "<xyz_ref>"
  Bus Selector1/1 -> Demux4/1  "<xyz>"
  Demux6/1 -> MATLAB Function2/10(vxr)
  Demux6/2 -> MATLAB Function2/11(vyr)
  statej/1 -> Bus Selector2/1
  Bus Selector2/1 -> Demux9/1, Demux1/1  "<xyz>"
  Demux4/1 -> MATLAB Function3/1(xi), MATLAB Function2/1(xi), MATLAB Function/1(xi)
  Demux4/2 -> MATLAB Function3/2(yi), MATLAB Function2/2(yi), MATLAB Function/2(yi)
  Demux1/1 -> MATLAB Function/7(xj)
  Demux1/2 -> MATLAB Function/8(yj)
  Bus Selector2/2 -> Demux8/1, Demux11/1  "<xyz_dot>"
  int1/1 -> MATLAB Function1/2(phiAlpha_int)
  MATLAB Function2/1(ui_gamma) -> MATLAB Function1/5(ui_gamma)
  statek/1 -> Bus Selector3/1
  Bus Selector3/2 -> Demux12/1, Demux13/1  "<xyz_dot>"
  Demux3/1 -> MATLAB Function/13(xk)
  Demux3/2 -> MATLAB Function/14(yk)
  Bus Selector3/1 -> Demux10/1, Demux3/1  "<xyz>"
  Demux9/1 -> MATLAB Function4/1(xj)
  Demux9/2 -> MATLAB Function4/2(yj)
  Demux10/1 -> MATLAB Function4/7(xk)
  Demux10/2 -> MATLAB Function4/8(yk)
  MATLAB Function/1(phiAlpha) -> int1/1, Scope1/1, MATLAB Function1/1(phiAlpha)
  Demux5/1 -> MATLAB Function2/7(xr)
  Demux5/2 -> MATLAB Function2/8(yr)
  Bus Selector1/2 -> Demux2/1  "<xyz_dot>"
  Demux4/3 -> MATLAB Function3/3(zi), MATLAB Function2/3(zi), MATLAB Function/3(zi)
  Demux3/3 -> MATLAB Function/15(zk)
  Demux5/3 -> MATLAB Function2/9(zr)
  Demux6/3 -> MATLAB Function2/12(vzr)
  MATLAB Function1/1(Ui) -> U_i/1
  Demux2/1 -> MATLAB Function/4(vxi), MATLAB Function2/4(vxi), MATLAB Function3/4(vxi)
  Demux2/2 -> MATLAB Function/5(vyi), MATLAB Function3/5(vyi), MATLAB Function2/5(vyi)
  Demux2/3 -> MATLAB Function/6(vzi), MATLAB Function3/6(vzi), MATLAB Function2/6(vzi)
  Demux1/3 -> MATLAB Function/9(zj)
  Demux11/1 -> MATLAB Function/10(vxj)
  Demux11/2 -> MATLAB Function/11(vyj)
  Demux11/3 -> MATLAB Function/12(vzj)
  Demux13/1 -> MATLAB Function/16(vxk)
  Demux13/2 -> MATLAB Function/17(vyk)
  Demux13/3 -> MATLAB Function/18(vzk)
  MATLAB Function/3(aive) -> MATLAB Function1/4(aive)
  Demux9/3 -> MATLAB Function4/3(zj)
  Demux10/3 -> MATLAB Function4/9(zk)
  MATLAB Function4/1(phiBetaniknei) -> Scope/1, MATLAB Function1/8(phiBetanei)
  Bus Selector/3 -> Terminator1/1  "<xyz_ref_ddot>"
  Demux8/1 -> MATLAB Function4/4(vxj)
  Demux8/2 -> MATLAB Function4/5(vyj)
  Demux8/3 -> MATLAB Function4/6(vzj)
  Demux12/1 -> MATLAB Function4/10(vxk)
  Demux12/2 -> MATLAB Function4/11(vyk)
  Demux12/3 -> MATLAB Function4/12(vzk)
  MATLAB Function4/2(bikve) -> MATLAB Function1/9(bikve)
  MATLAB Function3/1(phiBetanik) -> MATLAB Function1/6(phiBetak)
  MATLAB Function3/2(bikobs) -> MATLAB Function1/7(bikobs)
  MATLAB Function/2(aie) -> MATLAB Function1/3(aie)

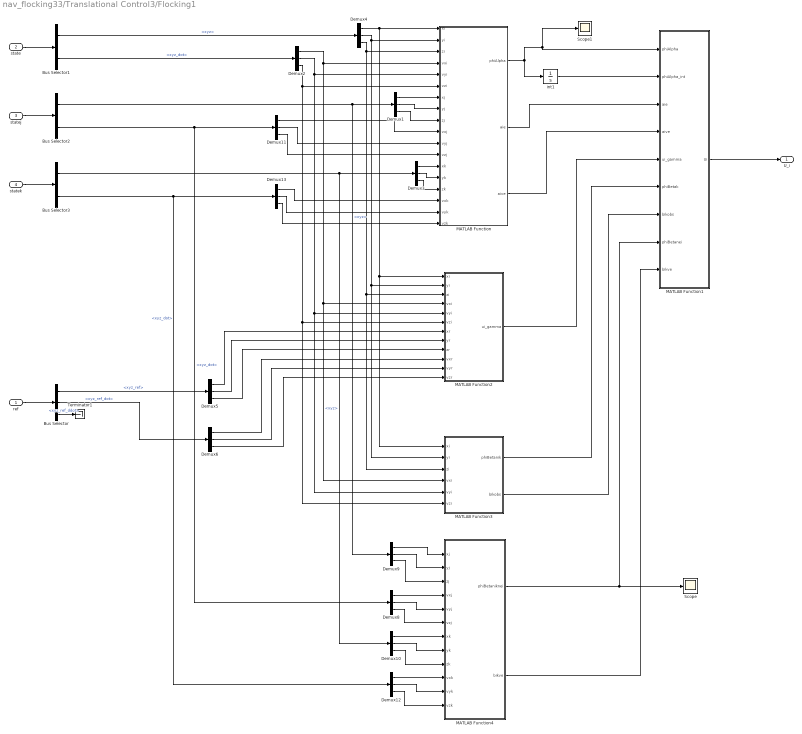
== system nav_flocking33/Translational Control3/Flocking1 ==
  ref : Inport
  state : Inport  Port=2
  statej : Inport  Port=3
  statek : Inport  Port=4
  Bus Selector : BusSelector  OutputSignals=xyz_ref,xyz_ref_dot,xyz_ref_ddot
  Bus Selector1 : BusSelector  OutputSignals=xyz,xyz_dot
  Bus Selector2 : BusSelector  OutputSignals=xyz,xyz_dot
  Bus Selector3 : BusSelector  OutputSignals=xyz,xyz_dot
  Demux{1..6,8..13} (12 alike) : Demux  Outputs=3
  MATLAB Function : MATLAB Function  TreatAsAtomicUnit=on
  MATLAB Function1 : MATLAB Function  TreatAsAtomicUnit=on
  MATLAB Function2 : MATLAB Function  TreatAsAtomicUnit=on
  MATLAB Function3 : MATLAB Function  TreatAsAtomicUnit=on
  MATLAB Function4 : MATLAB Function  TreatAsAtomicUnit=on
  Scope : Scope
  Scope1 : Scope
  Terminator1 : Terminator
  int1 : Integrator
  U_i : Outport  VectorParamsAs1DForOutWhenUnconnected=off
  wires:
  ref/1 -> Bus Selector/1
  state/1 -> Bus Selector1/1
  Bus Selector/2 -> Demux6/1  "<xyz_ref_dot>"
  Bus Selector/1 -> Demux5/1  "<xyz_ref>"
  Bus Selector1/1 -> Demux4/1  "<xyz>"
  Demux6/1 -> MATLAB Function2/10(vxr)
  Demux6/2 -> MATLAB Function2/11(vyr)
  statej/1 -> Bus Selector2/1
  Bus Selector2/1 -> Demux9/1, Demux1/1  "<xyz>"
  Demux4/1 -> MATLAB Function3/1(xi), MATLAB Function2/1(xi), MATLAB Function/1(xi)
  Demux4/2 -> MATLAB Function3/2(yi), MATLAB Function2/2(yi), MATLAB Function/2(yi)
  Demux1/1 -> MATLAB Function/7(xj)
  Demux1/2 -> MATLAB Function/8(yj)
  Bus Selector2/2 -> Demux8/1, Demux11/1  "<xyz_dot>"
  int1/1 -> MATLAB Function1/2(phiAlpha_int)
  MATLAB Function2/1(ui_gamma) -> MATLAB Function1/5(ui_gamma)
  statek/1 -> Bus Selector3/1
  Bus Selector3/2 -> Demux12/1, Demux13/1  "<xyz_dot>"
  Demux3/1 -> MATLAB Function/13(xk)
  Demux3/2 -> MATLAB Function/14(yk)
  Bus Selector3/1 -> Demux10/1, Demux3/1  "<xyz>"
  Demux9/1 -> MATLAB Function4/1(xj)
  Demux9/2 -> MATLAB Function4/2(yj)
  Demux10/1 -> MATLAB Function4/7(xk)
  Demux10/2 -> MATLAB Function4/8(yk)
  MATLAB Function/1(phiAlpha) -> int1/1, Scope1/1, MATLAB Function1/1(phiAlpha)
  Demux5/1 -> MATLAB Function2/7(xr)
  Demux5/2 -> MATLAB Function2/8(yr)
  Bus Selector1/2 -> Demux2/1  "<xyz_dot>"
  Demux4/3 -> MATLAB Function3/3(zi), MATLAB Function2/3(zi), MATLAB Function/3(zi)
  Demux3/3 -> MATLAB Function/15(zk)
  Demux5/3 -> MATLAB Function2/9(zr)
  Demux6/3 -> MATLAB Function2/12(vzr)
  MATLAB Function1/1(Ui) -> U_i/1
  Demux2/1 -> MATLAB Function/4(vxi), MATLAB Function2/4(vxi), MATLAB Function3/4(vxi)
  Demux2/2 -> MATLAB Function/5(vyi), MATLAB Function3/5(vyi), MATLAB Function2/5(vyi)
  Demux2/3 -> MATLAB Function/6(vzi), MATLAB Function3/6(vzi), MATLAB Function2/6(vzi)
  Demux1/3 -> MATLAB Function/9(zj)
  Demux11/1 -> MATLAB Function/10(vxj)
  Demux11/2 -> MATLAB Function/11(vyj)
  Demux11/3 -> MATLAB Function/12(vzj)
  Demux13/1 -> MATLAB Function/16(vxk)
  Demux13/2 -> MATLAB Function/17(vyk)
  Demux13/3 -> MATLAB Function/18(vzk)
  MATLAB Function/3(aive) -> MATLAB Function1/4(aive)
  Demux9/3 -> MATLAB Function4/3(zj)
  Demux10/3 -> MATLAB Function4/9(zk)
  MATLAB Function4/1(phiBetaniknei) -> Scope/1, MATLAB Function1/8(phiBetanei)
  Bus Selector/3 -> Terminator1/1  "<xyz_ref_ddot>"
  Demux8/1 -> MATLAB Function4/4(vxj)
  Demux8/2 -> MATLAB Function4/5(vyj)
  Demux8/3 -> MATLAB Function4/6(vzj)
  Demux12/1 -> MATLAB Function4/10(vxk)
  Demux12/2 -> MATLAB Function4/11(vyk)
  Demux12/3 -> MATLAB Function4/12(vzk)
  MATLAB Function4/2(bikve) -> MATLAB Function1/9(bikve)
  MATLAB Function3/1(phiBetanik) -> MATLAB Function1/6(phiBetak)
  MATLAB Function3/2(bikobs) -> MATLAB Function1/7(bikobs)
  MATLAB Function/2(aie) -> MATLAB Function1/3(aie)

== matlab function nav_flocking33/Dron_dynamics1/MATLAB Function1 ==
  data: X input; dX output; X2 input; dotq output; as input
function [dX,dotq] = fcn(X, X2, as)
% Jonatan Alvarez / October 2021
% Rotorcraft 3D Model (based on the quaternion parametrization) 

%Rotorcraft dimensions and parameters
m=0.65;   
g = 9.81;
Ix = 7.5e-3;
Iy = 7.5e-3;
Iz = 1.3e-2;
e  = 4.06e-6;
d  = 7.5e-7;
l  = (0.2)*(sin(pi/4));

%Inertia
Ii=[Ix 0 0; 0 Iy 0; 0 0 Iz];

%Extraction of data
x = X(1:3);
dx = X(4:6);
om = X(7:9); %Angular velocity

%Wind


%Separation of the angular velocity and quaternions in its components
om1 = om(1);
om2 = om(2);
om3 = om(3);

q = X2(1:4);
q1 = q(1);
q2 = q(2);
q3 = q(3);
q4 = q(4);
qv = [q2;q3;q4];

%EXTRACTION OF ROTOR SPEEDS AND FORCES COMPUTATION
u = as(1:4);
%Motor forces (e3)
f1= e*u(1)^2; f2=e*u(2)^2;  f3=e*u(3)^2; f4=e*u(4)^2; % rotors' blades lift forces
f1d = d*u(1)^2; f2d=d*u(2)^2;  f3d=d*u(3)^2; f4d=d*u(4)^2; %rotors' blades drag forces
%Torques
tau_phi = (1/sqrt(2))*l*(f1-f2-f3+f4) ;
tau_the = (1/sqrt(2))*l*(-f1-f2+f3+f4);
tau_psi = l*(f1d-f2d+f3d-f4d);
%MAIN Thrust and Torque vectors
Th =[0;0;f1+f2+f3+f4];
F = [tau_phi;tau_the;tau_psi];

%ROTATIONAL MOTION
%Quaternions
dq0 = 0.5*(-om1*q2 - om2*q3 - om3*q4);
dq1 = 0.5*(om1*q1 + om3*q3 - om2*q4);
dq2 = 0.5*(om2*q1 - om3*q2 + om1*q4);
dq3 = 0.5*(om3*q1 + om2*q2 - om1*q3);
%Attitude kinematics in quaternions
dotq = [dq0;dq1;dq2;dq3];  
%Attitude dynamics
dW =  inv(Ii)*( - cross(om,Ii*om) + F);

%TRANSLATIONAL MOTION
%Identity matrix
I3 = [1 0 0;
      0 1 0;
      0 0 1];
%Skew symmetrix matrix of vector part of the quaternion
sqv = [0 -q4 q3;
       q4 0 -q2;
       -q3 q2 0];
%Rotation matrix: given in Euler-Rodrigues formula
R = (q1^2 - qv'*qv)*I3 + 2*(qv*qv') - 2*q1*sqv;
%R = I3 - 2*q1*(sqv) + 2*(sqv)^2;
%Mass matrix
M_xi=[m  0  0;
      0  m  0;
      0  0  m];
%Vector fo Gravitational terms and thrust
G_xi=[0;0;m*g];
%Th = [0;0;T];
%Linear dynamics
Ddx =  inv(M_xi)*( -G_xi + R*Th);  % +fa

%Final vector
dX = [dx;Ddx;dW];

== matlab function nav_flocking33/Subsystem/Sliding mode (quaternions) ==
  data: qwe input; Gamma output; lam parameter; Ki parameter; K1 parameter; K2 parameter; aR parameter; s output
function [Gamma, s]  = fcn(qwe, lam, Ki, K1, K2, aR)

%Rotorcraft dimensions and parameters
Ix = 7.5e-3;
Iy = 7.5e-3;
Iz = 1.3e-2;

%Inertia
Ii=[Ix 0 0; 0 Iy 0; 0 0 Iz];

%Separation of rotational velocity and quaternion error in its components
qe = qwe(5:8);
qe1 = qe(1);
qe2 = qe(2);
qe3 = qe(3);
qe4 = qe(4);
qev = [qe2; qe3; qe4];

w = qwe(9:11);

iqe = qwe(12:15);
i_qe = [iqe(2); iqe(3); iqe(4)];

%Desired rotational velocity
wd = [0;0;0];

dwd = [0;0;0];

%Rotational velocity error in Euler
we = w - wd;
we1 = we(1);
we2 = we(2);
we3 = we(3);

%Quaternion error (derivative)
dqe0 = 0.5*(-we1*qe2 - we2*qe3 - we3*qe4);
dqe1 = 0.5*(we1*qe1 + we3*qe3 - we2*qe4);
dqe2 = 0.5*(we2*qe1 - we3*qe2 + we1*qe4);
dqe3 = 0.5*(we3*qe1 + we2*qe2 - we1*qe3);
dqe = [dqe1; dqe2; dqe3];

%Identity matrix
I3 = [1 0 0;
      0 1 0;
      0 0 1];
%Skew symmetrix matrix of vector part of the quaternion
sqev = [0 -qe4 qe3;
       qe4 0 -qe2;
       -qe3 qe2 0];
%ROTAION MATRIX: Given in Euler-Rodrigues formula
Re = (qe1^2 - qev'*qev)*I3 + 2*(qev*qev') - 2*qe1*sqev;

s = Ii*we + lam*qev + Ki*i_qe;

prod = cross(we,Re'*wd);

u = -lam*dqe - Ki*qev -Ii*(prod - Re'*dwd) + cross(w,Ii*w);       %Ks*qev

%Integral SMC 
Gamma = u - K1*tanh(inv(aR)*s) - K2*s;

== matlab function nav_flocking33/Translational Control3/Flocking1/MATLAB Function ==
  data: xi input; yi input; zi input; vxi input; vyi input; vzi input; phiAlpha output; aie output; aive output; xj input; yj input; zj input; vxj input; vyj input; vzj input; xk input; yk input; zk input; vxk input; vyk input; vzk input; epsilon parameter; a parameter; b parameter; c parameter; d parameter; e parameter; h parameter

function [phiAlpha, aie, aive]  = phiAlphaFcn(xi, yi, zi, vxi, vyi, vzi, xj, yj, zj, vxj, vyj, vzj, xk, yk, zk, vxk, vyk, vzk, epsilon, a, b, c, d, e, h)
    
    % Flocking parameters
    cAlpha = sigmaNormFun(c, epsilon) ;
    dAlpha = sigmaNormFun(d, epsilon) ;

    %%
    Pi = [xi;yi;zi] ;
    Pj = [xj;yj;zj] ;
    Pk = [xk;yk;zk] ;

    Vi = [vxi;vyi;vzi] ;
    Vj = [vxj;vyj;vzj] ;
    Vk = [vxk;vyk;vzk] ;
            
    %%
    sigmaNormj = sigmaNormFun(Pj - Pi, epsilon) ;
    nij = gradSigmaFun(Pj - Pi, epsilon) ;
    
    sigmaNormk = sigmaNormFun(Pk - Pi, epsilon) ;
    nik = gradSigmaFun(Pk - Pi, epsilon) ;

    %%
    sigma1j = sigma1Fun(sigmaNormj - dAlpha + e) ;
    sigma1k = sigma1Fun(sigmaNormk - dAlpha + e) ;
            
    %% Position
    phiAlphaj = 0.5 * bumpFcn(sigmaNormj/cAlpha,h) * ((a+b)*sigma1j + (a-b)) ;
    phiAlphanij = phiAlphaj.* nij ;
    
    phiAlphak = 0.5 * bumpFcn(sigmaNormk/cAlpha,h) * ((a+b)*sigma1k + (a-b)) ;
    phiAlphanik = phiAlphak.* nik ;

    phiAlpha = phiAlphanij + phiAlphanik;

    %
    aije = bumpFcn(sigmaNormj/cAlpha,h).*(Pj - Pi);

    aike = bumpFcn(sigmaNormj/cAlpha,h).*(Pk - Pi);

    aie = aije + aike;

    %% Velocity
    aijve = bumpFcn(sigmaNormj/cAlpha,h).*(Vj - Vi);

    aikve = bumpFcn(sigmaNormk/cAlpha,h).*(Vk - Vi);

    aive = aijve + aikve;
    
end

== matlab function nav_flocking33/Translational Control1/to_desired_angles ==
  data: Gamma input; cq_d output; Uz output
function [cq_d,Uz] = fcn(Gamma)

%Physical parameters
m = 0.65;
g = 9.81;

%Control signals separation
gamma = Gamma(1:3);
gamma1 = gamma(1);
gamma2 = gamma(2);
gamma3 = gamma(3);

%Desired Phi, theta, trust
psi = 0*pi/180;

phi = atan(gamma2/(gamma3+g));

theta = asin(-gamma1/(sqrt(gamma1^2+gamma2^2+(gamma3+g)^2)));

Uz = m*sqrt((gamma1)^2+(gamma2)^2+(gamma3+g)^2);

%Conversion to quaternions
q0 = cos(psi/2)*cos(theta/2)*cos(phi/2) + sin(psi/2)*sin(theta/2)*sin(phi/2);
q1 = cos(psi/2)*cos(theta/2)*sin(phi/2) - sin(psi/2)*sin(theta/2)*cos(phi/2);
q2 = cos(psi/2)*sin(theta/2)*cos(phi/2) + sin(psi/2)*cos(theta/2)*sin(phi/2);
q3 = sin(psi/2)*cos(theta/2)*cos(phi/2) - cos(psi/2)*sin(theta/2)*sin(phi/2);

cq_d = [q0;
        -q1;
        -q2;
        -q3];

== matlab function nav_flocking33/Dron_dynamics1/Mixer (Parrot ARDRONE) ==
  data: T input; w1 output size=1; tau input; w2 output size=1; w3 output size=1; w4 output size=1
function [w1,w2,w3,w4]   = fcn(T, tau)
%#codegen
tau_phi = tau(1); 
tau_the = tau(2); 
tau_psi = tau(3);

% This values vary in fonction of the geometry of the drone 
b= 4.06e-6;
d= 7.5e-7;
l= (0.2)*(sin(pi/4));

%Parrot AR-DRONE 
uT = T/b; 
uphi = (sqrt(2)*tau_phi)/(b*l);  
uthe = (sqrt(2)*tau_the)/(b*l);
upsi = tau_psi/(d*l);

%Mix by Motors
mixM1 = uT+uphi-uthe+upsi;  %uT + for all mixM
mixM2 = uT-uphi-uthe-upsi; 
mixM3 = uT-uphi+uthe+upsi; 
mixM4 = uT+uphi+uthe-upsi;

%rotors speeds [rads/s]
w1= sign(mixM1)*sqrt(abs((1/4)*mixM1));
w2= sign(mixM2)*sqrt(abs((1/4)*mixM2));
w3= sign(mixM3)*sqrt(abs((1/4)*mixM3));
w4= sign(mixM4)*sqrt(abs((1/4)*mixM4));

== matlab function nav_flocking33/Subsystem1/Sliding mode (quaternions) ==
  data: qwe input; Gamma output; lam parameter; Ki parameter; K1 parameter; K2 parameter; aR parameter; s output
function [Gamma, s]  = fcn(qwe, lam, Ki, K1, K2, aR)

%Rotorcraft dimensions and parameters
Ix = 7.5e-3;
Iy = 7.5e-3;
Iz = 1.3e-2;

%Inertia
Ii=[Ix 0 0; 0 Iy 0; 0 0 Iz];

%Separation of rotational velocity and quaternion error in its components
qe = qwe(5:8);
qe1 = qe(1);
qe2 = qe(2);
qe3 = qe(3);
qe4 = qe(4);
qev = [qe2; qe3; qe4];

w = qwe(9:11);

iqe = qwe(12:15);
i_qe = [iqe(2); iqe(3); iqe(4)];

%Desired rotational velocity
wd = [0;0;0];

dwd = [0;0;0];

%Rotational velocity error in Euler
we = w - wd;
we1 = we(1);
we2 = we(2);
we3 = we(3);

%Quaternion error (derivative)
dqe0 = 0.5*(-we1*qe2 - we2*qe3 - we3*qe4);
dqe1 = 0.5*(we1*qe1 + we3*qe3 - we2*qe4);
dqe2 = 0.5*(we2*qe1 - we3*qe2 + we1*qe4);
dqe3 = 0.5*(we3*qe1 + we2*qe2 - we1*qe3);
dqe = [dqe1; dqe2; dqe3];

%Identity matrix
I3 = [1 0 0;
      0 1 0;
      0 0 1];
%Skew symmetrix matrix of vector part of the quaternion
sqev = [0 -qe4 qe3;
       qe4 0 -qe2;
       -qe3 qe2 0];
%ROTAION MATRIX: Given in Euler-Rodrigues formula
Re = (qe1^2 - qev'*qev)*I3 + 2*(qev*qev') - 2*qe1*sqev;

s = Ii*we + lam*qev + Ki*i_qe;

prod = cross(we,Re'*wd);

u = -lam*dqe - Ki*qev -Ii*(prod - Re'*dwd) + cross(w,Ii*w);       %Ks*qev

%Integral SMC 
Gamma = u - K1*tanh(inv(aR)*s) - K2*s;

== matlab function nav_flocking33/Translational Control3/Flocking1/MATLAB Function1 ==
  data: phiAlpha input; phiAlpha_int input; aie input; aive input; ui_gamma input; phiBetak input; bikobs input; phiBetanei input; bikve input; Ui output size=3; KP parameter

function Ui  = ctrlLaw(phiAlpha, phiAlpha_int, aie, aive, ui_gamma, phiBetak, bikobs, phiBetanei, bikve, KP)  %, phiBetak, phiBetanei
    
    % Control gains and parameters
    Kx = KP(1); Ky = KP(2); Kz = KP(3);
    Kpx = KP(4); Kpy = KP(5); Kpz = KP(6);
    Kdx = KP(7); Kdy = KP(8); Kdz = KP(9);
    Kix = KP(10); Kiy = KP(11); Kiz = KP(12);
    cBetax = KP(13); cBetay = KP(14); cBetaz = KP(15);
    cdBetax = KP(16); cdBetay = KP(17); cdBetaz = KP(18);
    
        
    hx_dot = Kx * phiAlpha(1,1) + Kpx * aie(1,1) + Kdx * aive(1,1) + Kix * phiAlpha_int(1,1) + ui_gamma(1,1) + cBetax * (phiBetak(1,1) + phiBetanei(1,1)) + cdBetax * (bikobs(1,1) + bikve(1,1));
    hy_dot = Ky * phiAlpha(2,1) + Kpy * aie(2,1) + Kdy * aive(2,1) + Kiy * phiAlpha_int(2,1) + ui_gamma(2,1) + cBetay * (phiBetak(2,1) + phiBetanei(2,1)) + cdBetay * (bikobs(2,1) + bikve(2,1));
    hz_dot = Kz * phiAlpha(3,1) + Kpz * aie(3,1) + Kdz * aive(3,1) + Kiz * phiAlpha_int(3,1) + ui_gamma(3,1) + cBetaz * (phiBetak(3,1) + phiBetanei(3,1)) + cdBetaz * (bikobs(3,1) + bikve(3,1));
    

    Ui = [hx_dot; hy_dot; hz_dot] ;
        
end

== matlab function nav_flocking33/Translational Control2/to_desired_angles ==
  data: Gamma input; cq_d output; Uz output
function [cq_d,Uz] = fcn(Gamma)

%Physical parameters
m = 0.65;
g = 9.81;

%Control signals separation
gamma = Gamma(1:3);
gamma1 = gamma(1);
gamma2 = gamma(2);
gamma3 = gamma(3);

%Desired Phi, theta, trust
psi = 0*pi/180;

phi = atan(gamma2/(gamma3+g));

theta = asin(-gamma1/(sqrt(gamma1^2+gamma2^2+(gamma3+g)^2)));

Uz = m*sqrt((gamma1)^2+(gamma2)^2+(gamma3+g)^2);

%Conversion to quaternions
q0 = cos(psi/2)*cos(theta/2)*cos(phi/2) + sin(psi/2)*sin(theta/2)*sin(phi/2);
q1 = cos(psi/2)*cos(theta/2)*sin(phi/2) - sin(psi/2)*sin(theta/2)*cos(phi/2);
q2 = cos(psi/2)*sin(theta/2)*cos(phi/2) + sin(psi/2)*cos(theta/2)*sin(phi/2);
q3 = sin(psi/2)*cos(theta/2)*cos(phi/2) - cos(psi/2)*sin(theta/2)*sin(phi/2);

cq_d = [q0;
        -q1;
        -q2;
        -q3];

== matlab function nav_flocking33/Dron_dynamics2/MATLAB Function1 ==
  data: X input; dX output; X2 input; dotq output; as input
function [dX,dotq] = fcn(X, X2, as)
% Jonatan Alvarez / October 2021
% Rotorcraft 3D Model (based on the quaternion parametrization) 

%Rotorcraft dimensions and parameters
m=0.65;   
g = 9.81;
Ix = 7.5e-3;
Iy = 7.5e-3;
Iz = 1.3e-2;
e  = 4.06e-6;
d  = 7.5e-7;
l  = (0.2)*(sin(pi/4));

%Inertia
Ii=[Ix 0 0; 0 Iy 0; 0 0 Iz];

%Extraction of data
x = X(1:3);
dx = X(4:6);
om = X(7:9); %Angular velocity

%Wind


%Separation of the angular velocity and quaternions in its components
om1 = om(1);
om2 = om(2);
om3 = om(3);

q = X2(1:4);
q1 = q(1);
q2 = q(2);
q3 = q(3);
q4 = q(4);
qv = [q2;q3;q4];

%EXTRACTION OF ROTOR SPEEDS AND FORCES COMPUTATION
u = as(1:4);
%Motor forces (e3)
f1= e*u(1)^2; f2=e*u(2)^2;  f3=e*u(3)^2; f4=e*u(4)^2; % rotors' blades lift forces
f1d = d*u(1)^2; f2d=d*u(2)^2;  f3d=d*u(3)^2; f4d=d*u(4)^2; %rotors' blades drag forces
%Torques
tau_phi = (1/sqrt(2))*l*(f1-f2-f3+f4) ;
tau_the = (1/sqrt(2))*l*(-f1-f2+f3+f4);
tau_psi = l*(f1d-f2d+f3d-f4d);
%MAIN Thrust and Torque vectors
Th =[0;0;f1+f2+f3+f4];
F = [tau_phi;tau_the;tau_psi];

%ROTATIONAL MOTION
%Quaternions
dq0 = 0.5*(-om1*q2 - om2*q3 - om3*q4);
dq1 = 0.5*(om1*q1 + om3*q3 - om2*q4);
dq2 = 0.5*(om2*q1 - om3*q2 + om1*q4);
dq3 = 0.5*(om3*q1 + om2*q2 - om1*q3);
%Attitude kinematics in quaternions
dotq = [dq0;dq1;dq2;dq3];  
%Attitude dynamics
dW =  inv(Ii)*( - cross(om,Ii*om) + F);

%TRANSLATIONAL MOTION
%Identity matrix
I3 = [1 0 0;
      0 1 0;
      0 0 1];
%Skew symmetrix matrix of vector part of the quaternion
sqv = [0 -q4 q3;
       q4 0 -q2;
       -q3 q2 0];
%Rotation matrix: given in Euler-Rodrigues formula
R = (q1^2 - qv'*qv)*I3 + 2*(qv*qv') - 2*q1*sqv;
%R = I3 - 2*q1*(sqv) + 2*(sqv)^2;
%Mass matrix
M_xi=[m  0  0;
      0  m  0;
      0  0  m];
%Vector fo Gravitational terms and thrust
G_xi=[0;0;m*g];
%Th = [0;0;T];
%Linear dynamics
Ddx =  inv(M_xi)*( -G_xi + R*Th);  % +fa

%Final vector
dX = [dx;Ddx;dW];
